simulink library "Library_Betriebsstrategie"  (R2018b)
settings: Solver=VariableStepAuto  StartTime=0.0  StopTime=10.0  RelTol=1e-3  EnableMultiTasking=on
undefined symbols (not defined in the file): akt_eUELG_HA, akt_eUELG_VA, akt_keinMVS_HA, akt_keinMVS_VA, akt_LSD_HA, akt_LSD_VA, akt_mUELG_HA, akt_mUELG_VA, akt_OD_HA, akt_OD_VA, DiscIntNeverNeededParam, magnitude, mu_road, mu_road_LF, mu_road_LR, mu_road_RF, mu_road_RR, par_MDT, par_VEH, stepsize
libraries: simulink x13
(part 1 of 6)
settings Model: Creator=ga76fur  LastModifiedBy=ga35gug
settings DataIOCC: LimitDataPoints=on
settings OptimizationCC: LifeSpan=inf
settings DebuggingCC: AllowSymbolicDim=off  SFUnexpectedBacktrackingDiag=warning  SFNoUnconditionalDefaultTransitionDiag=warning  SFExecutionAtInitializationDiag=none
settings ModelReferenceCC: PropagateSignalLabelsOutOfModel=off
settings SFSimCC: SimUseLocalCustomCode=off
settings RTWCC: RTWUseLocalCustomCode=off
settings CodeAppCC: StateflowObjectComments=on
settings GRTTargetCC: TargetLangStandard=C89/C90 (ANSI)
settings ConfigComp: CovMetricSettings=dw  CovHtmlReporting=on  CovSaveCumulativeToWorkspaceVar=on  CovSaveSingleToWorkspaceVar=on  CovExternalEMLEnable=off

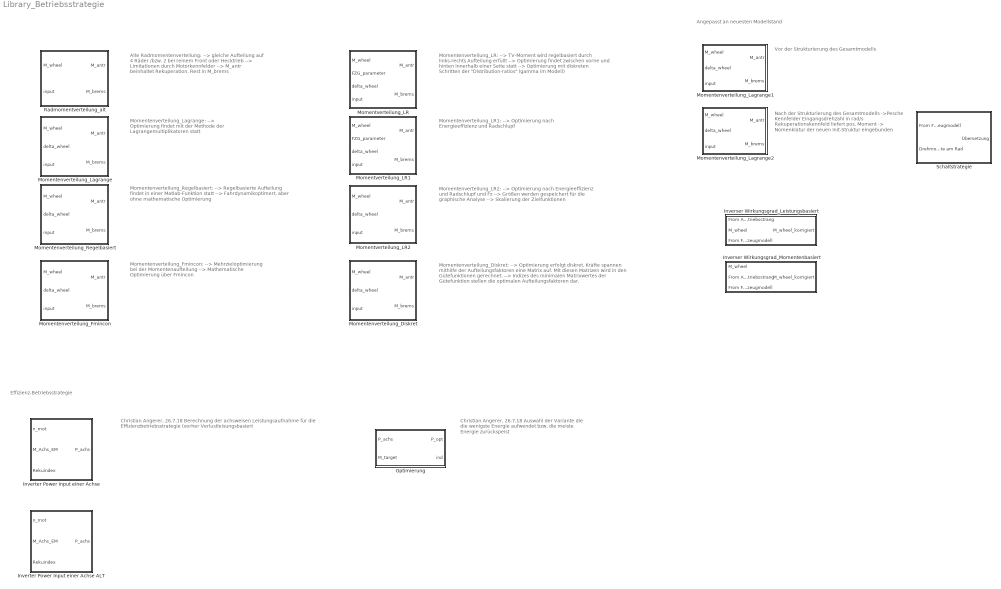
== system Library_Betriebsstrategie ==
  note: Effizienz-Betriebsstrategie
  note: Christian Angerer, 26.7.18
      | Berechnung der achsweisen Leistungsaufnahme für die Effizienzbetriebsstrategie
      | (vorher Verlustleisungsbasiert
  note: Nach der Strukturierung des Gesamtmodells
      | ->Pesche Kennfelder
      | 	Eingangsdrehzahl in rad/s
      | 	Rekuperationskennfeld liefert pos. Moment
      | -> Nomenklatur der neuen Init-Struktur eingebunden
  note: Vor der Strukturierung des Gesamtmodells
  note: Angepasst an neuesten Modellstand
  note: Momentenverteilung_Lagrange:
      | --> Optimierung findet mit der Methode der
      | 	Lagrangemultiplikatoren statt
  note: Momentenverteilung_LR1:
      | --> Optimierung nach Energieeffizienz und Radschlupf
  note: Momentenverteilung_Diskret:
      | --> Optimierung erfolgt diskret. Kräfte spannen mithilfe der
      | 	Aufteilungsfaktoren eine Matrix auf. Mit diesen Matrizen wird in den 		Gütefunktionen gerechnet.
      | --> Indizes des minimalen Matrixwertes der Gütefunktion stellen die 			optimalen Aufteilungsfaktoren dar.
  note: Momentenverteilung_Fmincon:
      | --> Mehrzieloptimierung bei der Momentenaufteilung
      | --> Mathematische Optimierung über Fmincon
  note: Momentenverteilung_Regelbasiert:
      | --> Regelbasierte Aufteilung findet in einer Matlab-Funktion statt
      | --> Fahrdynamikoptimert, aber ohne mathematische Optimierung
  note: Momentenverteilung_LR:
      | --> TV-Moment wird regelbasiert durch links-rechts Aufteilung erfüllt
      | --> Optimierung findet zwischen vorne und hinten
      | innerhalb einer Seite statt
      | --> Optimierung mit diskreten Schritten der "Distribution-ratios"
      | (gamma im Modell)
  note: Alte Radmomentenverteilung:
      | --> gleiche Aufteilung auf 4 Räder
      |     /bzw. 2 bei reinem Front oder Hecktrieb
      | --> Limitationen durch Motorkennfelder
      | --> M_antr beinhaltet Rekuperation, Rest in M_brems
  note: Momentenverteilung_LR2:
      | --> Optimierung nach Energieeffizienz und Radschlupf und Fz
      | --> Größen werden gespeichert für die graphische Analyse
      | --> Skalierung der Zielfunktionen
  note: Christian Angerer, 26.7.18
      | Auswahl der Variante die die wenigste Energie
      | aufwendet bzw. die meiste Energie zurückspeist
  Inverser Wirkungsgrad_Leistungsbasiert : Subsystem
  Inverser Wirkungsgrad_Momentenbasiert : Subsystem
  Inverter Power Input einer Achse : Subsystem  mask{U_RMS=par_MDT.VA.em.U_RMS, az=par_MDT.AUS.akt.az_VA, Powerfactor_map=par_MDT.VA.inv.Powerfactor_map, torque=par_MDT.VA.inv.torque, speed=par_MDT.VA.inv.speed, efficiency_map_LE=par_MDT.VA.inv.efficiency_map.efficiency_map_LE, current=par_MDT.VA.inv.current, voltage=par_MDT.VA.inv.voltage, powerfactor=par_MDT.VA.inv.powerfactor, MotorEffMap3D=par_MDT.VA.em.MotorEffMap3D, MotorEffMap3D_w=par_MDT.VA.em.MotorEffMap3D_w, MotorEffMap3D_M=par_MDT.VA.em.MotorEffMap3D_M, GeneratorEffMap3D=par_MDT.VA.em.GeneratorEffMap3D, GeneratorEffMap3D_w=par_MDT.VA.em.GeneratorEffMap3D_w, GeneratorEffMap3D_M=par_MDT.VA.em.GeneratorEffMap3D_M}
      mask prompts: U_RMS "RMS-Spannung"; az "Achszentrale Konfiguration"; Powerfactor_map "Map"; torque "torque-vector"; speed "speed-vector"; efficiency_map_LE "Map"; current "Stromvektor"; voltage "Spannungsvektor"; powerfactor "Powerfactor-Vektor"; MotorEffMap3D "Map"; MotorEffMap3D_w "Omega-Vektor"; MotorEffMap3D_M "Momenten-Vektor"; GeneratorEffMap3D "Map"; GeneratorEffMap3D_w "Omega-Vektor"; GeneratorEffMap3D_M "Momenten-Vektor"
      mask DialogControl Container3 Prompt: Einzelwerte
      mask DialogControl ParameterGroupVar Prompt: Powerfactor-Map
      mask DialogControl Container4 Prompt: LE-Efficiency Map
      mask DialogControl Container5 Prompt: Motor-Efficiency Maps
      mask DialogControl Container6 Prompt: Gen-Efficiency Maps
  Inverter Power Input einer Achse ALT : Subsystem  mask{U_RMS=par_MDT.VA.em.U_RMS, az=par_MDT.AUS.akt.az_VA, Powerfactor_map=par_MDT.VA.inv.Powerfactor_map, torque=par_MDT.VA.inv.torque, speed=par_MDT.VA.inv.speed, efficiency_map_LE=par_MDT.VA.inv.efficiency_map.efficiency_map_LE, current=par_MDT.VA.inv.current, voltage=par_MDT.VA.inv.voltage, powerfactor=par_MDT.VA.inv.powerfactor, MotorEffMap3D=par_MDT.VA.em.MotorEffMap3D, MotorEffMap3D_w=par_MDT.VA.em.MotorEffMap3D_w, MotorEffMap3D_M=par_MDT.VA.em.MotorEffMap3D_M, GeneratorEffMap3D=par_MDT.VA.em.GeneratorEffMap3D, GeneratorEffMap3D_w=par_MDT.VA.em.GeneratorEffMap3D_w, GeneratorEffMap3D_M=par_MDT.VA.em.GeneratorEffMap3D_M}
      mask prompts: U_RMS "RMS-Spannung"; az "Achszentrale Konfiguration"; Powerfactor_map "Map"; torque "torque-vector"; speed "speed-vector"; efficiency_map_LE "Map"; current "Stromvektor"; voltage "Spannungsvektor"; powerfactor "Powerfactor-Vektor"; MotorEffMap3D "Map"; MotorEffMap3D_w "Omega-Vektor"; MotorEffMap3D_M "Momenten-Vektor"; GeneratorEffMap3D "Map"; GeneratorEffMap3D_w "Omega-Vektor"; GeneratorEffMap3D_M "Momenten-Vektor"
      mask DialogControl Container3 Prompt: Einzelwerte
      mask DialogControl ParameterGroupVar Prompt: Powerfactor-Map
      mask DialogControl Container4 Prompt: LE-Efficiency Map
      mask DialogControl Container5 Prompt: Motor-Efficiency Maps
      mask DialogControl Container6 Prompt: Gen-Efficiency Maps
  Momentenverteilung_Diskret : Subsystem
  Momentenverteilung_Fmincon : Subsystem
  Momentenverteilung_Lagrange : Subsystem
  Momentenverteilung_Lagrange1 : Subsystem
  Momentenverteilung_Lagrange2 : Subsystem
  Momentenverteilung_Regelbasiert : Subsystem
  Momentverteilung_LR : Subsystem
  Momentverteilung_LR1 : Subsystem
  Momentverteilung_LR2 : Subsystem
  Optimierung : MATLAB Function  TreatAsAtomicUnit=on
  Radmomentverteilung_alt : Subsystem
  Schaltstrategie : Subsystem

== system Library_Betriebsstrategie/Inverser Wirkungsgrad_Leistungsbasiert ==
  note: Das Modell berücksichtigt nun einen verlustbehafteten Antriebsstrang vor dem Fahrzeugmodell.
      | --> Der Inverse Gesamtwirkungsgrad des vorherigen Zeitschrittes wird auf das Gesamtwunschmoment aufmultipliziert.
      | eta=P_ab/(P_ab+P_v)
  From Antriebsstrang : Inport
  M_wheel : Inport  Port=2
  From Fahrzeugmodell : Inport  Port=3
  1 : Constant
  Abs : Abs
  Abs1 : Abs
  Add : Sum
  Divide : Product  Inputs=/*
  Divide1 : Product  Inputs=/*
  Eins : Constant
  Memory : Memory
  Memory1 : Memory
  Product : Product
  Scope : Scope  NumInputPorts=2
  Scope1 : Scope  NumInputPorts=2
  Switch : Switch  Criteria=u2 > Threshold  Threshold=0.1
  M_wheel_korrigiert : Outport
  wires:
  Product/1 -> Scope1/1, M_wheel_korrigiert/1
  Eins/1 -> Divide/2
  Add/1 -> Switch/2, Divide1/1
  From Antriebsstrang/1 -> Scope/1, Memory/1
  Divide1/1 -> Divide/1
  Memory/1 -> Abs/1
  Memory1/1 -> Abs1/1
  Divide/1 -> Switch/1
  M_wheel/1 -> Scope1/2, Product/2
  Switch/1 -> Product/1
  1/1 -> Switch/3
  Abs/1 -> Add/1
  Abs1/1 -> Add/2, Divide1/2
  From Fahrzeugmodell/1 -> ?
  ? -> Scope/2, Memory1/1

== system Library_Betriebsstrategie/Inverser Wirkungsgrad_Momentenbasiert ==
  M_wheel : Inport
  From Antriebsstrang : Inport  Port=2
  From Fahrzeugmodell : Inport  Port=3
  1 : Constant
  Abs : Abs
  Abs1 : Abs
  Add1 : Sum  Inputs=++++
  Divide : Product  Inputs=/*
  Memory : Memory
  Memory1 : Memory
  Product : Product
  Scope : Scope  NumInputPorts=2
  Scope1 : Scope  NumInputPorts=2
  Switch : Switch  Criteria=u2 > Threshold
  M_wheel_korrigiert : Outport
  wires:
  Product/1 -> Scope/1, M_wheel_korrigiert/1
  M_wheel/1 -> Scope1/1, Memory1/1, Scope/2, Product/2
  Add1/1 -> Scope1/2, Memory/1
  Memory/1 -> Abs/1
  Memory1/1 -> Abs1/1
  Switch/1 -> Product/1
  1/1 -> Switch/3
  Abs1/1 -> Divide/2
  From Antriebsstrang/1 -> ?
  ? -> Add1/1
  ? -> Add1/2
  ? -> Add1/3
  ? -> Add1/4
  Abs/1 -> Switch/2, Divide/1
  Divide/1 -> Switch/1

== system Library_Betriebsstrategie/Inverter Power Input einer Achse ==
  note: Luca Mantovani, 05.9.18
      | Power estimation for electronics and motor is calculated with the same logic as found in Antriebsstrang una Radmomentverteilung. The electric power entering the motor is evaluated first and with the result the power at battery level is found.
  n_mot : Inport
  M_Achs_EM : Inport  Port=2
  Rekuindex : Inport  Port=3
  Abs{1..2,4..6} (5 alike) : Abs
  Constant1 : Constant  Value=U_RMS
  "Falls radnahe Maschine " : Subsystem
  Falls radnahe Maschine 1 : Subsystem
  Gain : Gain  Gain=-1
  Gain2 : Gain  Gain=-1
  Math Function : Math  Operator=pow  SaturateOnIntegerOverflow=on
  Math Function1 : Math  Operator=pow  SaturateOnIntegerOverflow=on
  Powerfactorberechnung : Subsystem
  Product1 : Product  Inputs=**
  Product3 : Product  Inputs=**
  Product5 : Product  Inputs=**
  Sign : Signum
  Stromberechnung : Subsystem
  W-->kW : Gain  Gain=0.001
  Wirkungsgradberechnung : Subsystem
  Wirkungsgradberechnung1 : Subsystem
  P_achs : Outport
  wires:
  Product1/1 -> Product3/1
  Abs6/1 -> Falls radnahe Maschine 1/1(M_achs_EM)
  W-->kW/1 -> P_achs/1
  Math Function/1 -> Product3/2
  Product5/1 -> Abs6/1  "P_inverter"
  M_Achs_EM/1 -> "Falls radnahe Maschine "/1(M_achs_EM)
  Product3/1 -> Abs2/1, Sign/1, Product5/2  "P_EM"
  Gain/1 -> Math Function/2
  Wirkungsgradberechnung/1(Wirkungsgrad EM) -> Math Function/1
  Rekuindex/1 -> Gain/1
  "Falls radnahe Maschine "/1(M_mot) -> Product1/2, Abs4/1, Wirkungsgradberechnung/2(M_mot)
  Abs2/1 -> Stromberechnung/1(Leistung)
  Wirkungsgradberechnung1/1(Wirkungsgrad_LE) -> Math Function1/1
  Abs5/1 -> Powerfactorberechnung/2(Drehzahl)
  Abs4/1 -> Powerfactorberechnung/1(Drehmoment)
  Powerfactorberechnung/1(Powerfactor) -> Stromberechnung/3(Powerfactor), Wirkungsgradberechnung1/3(Powerfactor)
  n_mot/1 -> Product1/1, Abs1/1, Abs5/1
  Sign/1 -> Gain2/1
  Gain2/1 -> Math Function1/2
  Constant1/1 -> Stromberechnung/2(Spannung), Wirkungsgradberechnung1/2(Spannung)
  Stromberechnung/1(Strom) -> Wirkungsgradberechnung1/1(Strom)
  Math Function1/1 -> Product5/1
  Abs1/1 -> Wirkungsgradberechnung/1(n_mot)
  Falls radnahe Maschine 1/1(M_mot) -> W-->kW/1

== system Library_Betriebsstrategie/Inverter Power Input einer Achse ALT ==
  n_mot : Inport
  M_Achs_EM : Inport  Port=2
  Rekuindex : Inport  Port=3
  Abs : Abs
  Abs6 : Abs
  Add1 : Sum
  Constant2 : Constant  Value=U_RMS
  "Falls radnahe Maschine " : Subsystem
  Leistungselektronik : Subsystem
  Product1 : Product  Inputs=**
  Product3 : Product  Inputs=**
  Product5 : Product  Inputs=**
  W-->kW : Gain  Gain=0.001
  Wirkungsgradberechnung : Subsystem
  P_achs : Outport
  wires:
  Product1/1 -> Product3/1, Product5/2
  Abs/1 -> Add1/2
  Abs6/1 -> Add1/1
  Add1/1 -> W-->kW/1
  W-->kW/1 -> P_achs/1
  Constant2/1 -> Leistungselektronik/1(RMS Spannung)
  "Falls radnahe Maschine "/1(M_mot) -> Leistungselektronik/2(Drehmoment_1EM), Wirkungsgradberechnung/2(M_mot)
  Wirkungsgradberechnung/1(Wirkungsgrad EM) -> Product3/2
  Leistungselektronik/1(Verlustgrad LE) -> Product5/1
  Rekuindex/1 -> Wirkungsgradberechnung/3(Rekuindex)
  Product5/1 -> Abs6/1  "P_loss_inverter"
  Product3/1 -> Abs/1  "P_EM"
  M_Achs_EM/1 -> "Falls radnahe Maschine "/1(M_achs_EM), Product1/2
  n_mot/1 -> Product1/1, Wirkungsgradberechnung/1(n_mot), Leistungselektronik/3("Drehzahl ")

== system Library_Betriebsstrategie/Momentenverteilung_Diskret ==
  M_wheel : Inport
  delta_wheel : Inport  Port=2
  input : Inport  Port=3
  Bus Selector3 : BusSelector  OutputSignals=x.vx
  Constant1 : Constant  Value=par_VEH.bkv
  Feedback Controller : Subsystem
  Gierrate Referenz Berechnung : Subsystem
  Memory : Memory
  Momente für die Reibbremse : Subsystem
  Radmomentenaufteilung : Subsystem
  Scope : Scope  NumInputPorts=2
  M_antr : Outport
  M_brems : Outport  Port=2
  wires:
  delta_wheel/1 -> Gierrate Referenz Berechnung/2(delta_wheel)
  input/1 -> Memory/1
  Feedback Controller/1(M_z_desired) -> Radmomentenaufteilung/2(M_z_desired), Scope/1  "M_z_desired"
  Gierrate Referenz Berechnung/1(Gierrate ref) -> Feedback Controller/2(Gierrate ref)  "psip_ref"
  Radmomentenaufteilung/1(M_antr) -> M_antr/1, Momente für die Reibbremse/1(M_antr)
  Momente für die Reibbremse/1(M_brems) -> M_brems/1
  M_wheel/1 -> Momente für die Reibbremse/2(M_wheel), Radmomentenaufteilung/3(M_wheel), Scope/2
  Bus Selector3/1 -> Momente für die Reibbremse/3(v_x)  "<vx>"
  Memory/1 -> Gierrate Referenz Berechnung/1(input), Feedback Controller/1(Input), Radmomentenaufteilung/1(Input), Bus Selector3/1
  Constant1/1 -> Momente für die Reibbremse/4(bkv)

== system Library_Betriebsstrategie/Momentenverteilung_Fmincon ==
  M_wheel : Inport
  delta_wheel : Inport  Port=2
  input : Inport  Port=3
  Bus Selector3 : BusSelector  OutputSignals=x.vx
  Constant1 : Constant  Value=par_VEH.bkv
  Feedback Controller : Subsystem
  Gierrate Referenz Berechnung : Subsystem
  Limitierungen gesamt : Subsystem
  Memory : Memory
  Momente für die Reibbremse : Subsystem
  Motor Limits : Subsystem
  Radmomentenaufteilung : Subsystem
  Reifen Limits : Subsystem
  M_antr : Outport
  M_brems : Outport  Port=2
  wires:
  delta_wheel/1 -> Gierrate Referenz Berechnung/2(delta_wheel)
  input/1 -> Memory/1
  Feedback Controller/1(M_z_desired) -> Radmomentenaufteilung/3(M_z_desired)  "M_z_desired"
  Gierrate Referenz Berechnung/1(Gierrate ref) -> Feedback Controller/2(Gierrate ref)  "psip_ref"
  Radmomentenaufteilung/1(M_antr) -> M_antr/1, Momente für die Reibbremse/1(M_antr)
  Momente für die Reibbremse/1(M_brems) -> M_brems/1
  M_wheel/1 -> Momente für die Reibbremse/2(M_wheel), Radmomentenaufteilung/4(M_wheel)
  Bus Selector3/1 -> Momente für die Reibbremse/3(v_x)  "<vx>"
  Reifen Limits/1(Fx_limit) -> Limitierungen gesamt/1(Fx_limit)
  Motor Limits/1(M_limit) -> Limitierungen gesamt/2(M_limit)
  Memory/1 -> Reifen Limits/1(Input), Motor Limits/1(Input), Feedback Controller/1(Input), Bus Selector3/1, Radmomentenaufteilung/2(Input), Gierrate Referenz Berechnung/1(input)
  Limitierungen gesamt/1(Fx_limits) -> Radmomentenaufteilung/1(Fx_limits)
  Constant1/1 -> Momente für die Reibbremse/4(bkv)

== system Library_Betriebsstrategie/Momentenverteilung_Lagrange ==
  M_wheel : Inport
  delta_wheel : Inport  Port=2
  input : Inport  Port=3
  Bus Selector3 : BusSelector  OutputSignals=x.vx
  Feedback Controller : Subsystem
  Gierrate Referenz Berechnung : Subsystem
  Memory : Memory
  Momente für die Reibbremse : Subsystem
  Radmomentenaufteilung : Subsystem
  M_antr : Outport
  M_brems : Outport  Port=2
  wires:
  delta_wheel/1 -> Gierrate Referenz Berechnung/2(delta_wheel), Radmomentenaufteilung/4(Delta_wheel)
  input/1 -> Memory/1
  Feedback Controller/1(M_z_desired) -> Radmomentenaufteilung/2(M_z_desired)  "M_z_desired"
  Gierrate Referenz Berechnung/1(Gierrate ref) -> Feedback Controller/2(Gierrate ref)  "psip_ref"
  Radmomentenaufteilung/1(M_antr) -> M_antr/1, Momente für die Reibbremse/1(M_antr)
  Momente für die Reibbremse/1(M_brems) -> M_brems/1
  M_wheel/1 -> Momente für die Reibbremse/2(M_wheel), Radmomentenaufteilung/3(M_wheel)
  Bus Selector3/1 -> Momente für die Reibbremse/3(v_x)  "<vx>"
  Memory/1 -> Feedback Controller/1(Input), Bus Selector3/1, Radmomentenaufteilung/1(Input), Gierrate Referenz Berechnung/1(input)

== system Library_Betriebsstrategie/Momentenverteilung_Lagrange1 ==
  M_wheel : Inport
  delta_wheel : Inport  Port=2
  input : Inport  Port=3
  Bus Selector3 : BusSelector  OutputSignals=x.vx
  Feedback Controller : Subsystem
  Gierrate Referenz Berechnung : Subsystem
  Limitierungen gesamt (mit MVS Limits) : Subsystem
  Memory : Memory
  Momente für die Reibbremse : Subsystem
  Motor Limits : Subsystem
  Radmomentenaufteilung : Subsystem
  Reifen Limits : Subsystem
  Scope : Scope  NumInputPorts=2
  M_antr : Outport
  M_brems : Outport  Port=2
  wires:
  Bus Selector3/1 -> Momente für die Reibbremse/3(v_x)  "<vx>"
  M_wheel/1 -> Radmomentenaufteilung/4(M_wheel), Momente für die Reibbremse/2(M_wheel), Scope/2
  Momente für die Reibbremse/1(M_brems) -> M_brems/1
  Radmomentenaufteilung/1(M_antr) -> M_antr/1, Momente für die Reibbremse/1(M_antr)
  Gierrate Referenz Berechnung/1(Gierrate ref) -> Feedback Controller/2(Gierrate ref)  "psip_ref"
  Feedback Controller/1(M_z_desired) -> Radmomentenaufteilung/3(M_z_desired), Scope/1  "M_z_desired"
  input/1 -> Memory/1
  delta_wheel/1 -> Radmomentenaufteilung/5(Delta_wheel), Gierrate Referenz Berechnung/2(delta_wheel)
  Motor Limits/2(M_limit_zentral) -> Limitierungen gesamt (mit MVS Limits)/3(M_limit_zentral)
  Memory/1 -> Gierrate Referenz Berechnung/1(input), Bus Selector3/1, Radmomentenaufteilung/2(Input), Feedback Controller/1(Input), Motor Limits/1(Input), Reifen Limits/1(Input)
  Motor Limits/1(M_limit) -> Limitierungen gesamt (mit MVS Limits)/2(M_limit)
  Reifen Limits/1(Fx_limit) -> Limitierungen gesamt (mit MVS Limits)/1(Fx_limit)
  Limitierungen gesamt (mit MVS Limits)/1(Fx_limits) -> Radmomentenaufteilung/1(Fx_limits)

== system Library_Betriebsstrategie/Momentenverteilung_Lagrange2 ==
  M_wheel : Inport
  delta_wheel : Inport  Port=2
  input : Inport  Port=3
  Bus Selector3 : BusSelector  OutputSignals=x.vx
  Feedback Controller : Subsystem
  Gierrate Referenz Berechnung : Subsystem
  Limitierungen gesamt (mit MVS Limits) : Subsystem
  Memory : Memory
  Momente für die Reibbremse : Subsystem
  Motor Limits : Subsystem
  Radmomentenaufteilung1 : Subsystem
  Reifen Limits : Subsystem
  Scope : Scope  NumInputPorts=2
  M_antr : Outport
  M_brems : Outport  Port=2
  wires:
  Limitierungen gesamt (mit MVS Limits)/1(Fx_limits) -> Radmomentenaufteilung1/1(Fx_limits)
  Reifen Limits/1(Fx_limit) -> Limitierungen gesamt (mit MVS Limits)/1(Fx_limit)
  Motor Limits/1(M_limit) -> Limitierungen gesamt (mit MVS Limits)/2(M_limit)
  Memory/1 -> Motor Limits/1(Input), Reifen Limits/1(Input), Feedback Controller/1(Input), Bus Selector3/1, Radmomentenaufteilung1/2(Input), Gierrate Referenz Berechnung/1(input)
  Motor Limits/2(M_limit_zentral) -> Limitierungen gesamt (mit MVS Limits)/3(M_limit_zentral)
  delta_wheel/1 -> Radmomentenaufteilung1/5(Delta_wheel), Gierrate Referenz Berechnung/2(delta_wheel)
  input/1 -> Memory/1
  Feedback Controller/1(M_z_desired) -> Radmomentenaufteilung1/3(M_z_desired), Scope/1  "M_z_desired"
  Gierrate Referenz Berechnung/1(Gierrate ref) -> Feedback Controller/2(Gierrate ref)  "psip_ref"
  Radmomentenaufteilung1/1(M_antr) -> M_antr/1, Momente für die Reibbremse/1(M_antr)
  Momente für die Reibbremse/1(M_brems) -> M_brems/1
  M_wheel/1 -> Scope/2, Radmomentenaufteilung1/4(M_wheel), Momente für die Reibbremse/2(M_wheel)
  Bus Selector3/1 -> Momente für die Reibbremse/3(v_x)  "<vx>"

== system Library_Betriebsstrategie/Momentenverteilung_Regelbasiert ==
  M_wheel : Inport
  delta_wheel : Inport  Port=2
  input : Inport  Port=3
  Bus Selector3 : BusSelector  OutputSignals=x.vx
  Constant10 : Constant  Value=par_VEH.bkv
  Feedback Controller : Subsystem
  Gierrate Referenz Berechnung : Subsystem
  Limitierungen gesamt : Subsystem
  Memory : Memory
  Momente für die Reibbremse : Subsystem
  Motor Limits : Subsystem
  Radmomentenaufteilung : Subsystem
  Reifen Limits : Subsystem
  M_antr : Outport
  M_brems : Outport  Port=2
  wires:
  delta_wheel/1 -> Gierrate Referenz Berechnung/2(delta_wheel)
  input/1 -> Memory/1
  Feedback Controller/1(M_z_desired) -> Radmomentenaufteilung/4(M_z_desired)  "M_z_desired"
  Gierrate Referenz Berechnung/1(Gierrate ref) -> Feedback Controller/2(Gierrate ref)  "psip_ref"
  Radmomentenaufteilung/1(M_antr) -> Momente für die Reibbremse/1(M_antr), M_antr/1
  Momente für die Reibbremse/1(M_brems) -> M_brems/1
  M_wheel/1 -> Momente für die Reibbremse/2(M_wheel), Radmomentenaufteilung/3(M_wheel)
  Bus Selector3/1 -> Momente für die Reibbremse/3(v_x)  "<vx>"
  Memory/1 -> Gierrate Referenz Berechnung/1(input), Reifen Limits/1(Input), Motor Limits/1(Input), Feedback Controller/1(Input), Bus Selector3/1, Radmomentenaufteilung/2(Input)
  Motor Limits/1(M_limit) -> Limitierungen gesamt/2(M_limit)
  Limitierungen gesamt/1(Fx_limits) -> Radmomentenaufteilung/1(Fx_limits)
  Constant10/1 -> Momente für die Reibbremse/4(bkv)
  Reifen Limits/1(Fx_limit) -> Limitierungen gesamt/1(Fx_limit)

== system Library_Betriebsstrategie/Momentverteilung_LR ==
  M_wheel : Inport
  FZG_parameter : Inport  Port=2
  delta_wheel : Inport  Port=3
  input : Inport  Port=4
  Bus Creator : BusCreator  Inputs=4
  Bus Creator1 : BusCreator  Inputs=4
  Bus Selector1 : BusSelector  OutputSignals=Iz
  Bus Selector2 : BusSelector  OutputSignals=psi.psip
  Bus Selector3 : BusSelector  OutputSignals=x.vx
  Bus Selector4 : BusSelector  OutputSignals=bkv
  Feedback Controller : Subsystem
  Gierrate Referenz Berechnung : Subsystem
  Memory : Memory
  Momente für die Reibbremse : Subsystem
  Motor Limits : Subsystem
  Radmomentenaufteilung : Subsystem
  Reifen Limits : Subsystem
  M_antr : Outport
  M_brems : Outport  Port=2
  wires:
  FZG_parameter/1 -> Bus Selector1/1, Radmomentenaufteilung/4(FZG parameter), Bus Selector4/1, Gierrate Referenz Berechnung/3(FZG parameter)
  delta_wheel/1 -> Gierrate Referenz Berechnung/2(delta_wheel)
  input/1 -> Memory/1
  Feedback Controller/1(M_z_desired) -> Radmomentenaufteilung/3(M_z_desired)  "M_z_desired"
  Gierrate Referenz Berechnung/1(Gierrate ref) -> Feedback Controller/2(Gierrate ref)  "psip_ref"
  Bus Selector2/1 -> Feedback Controller/1(Gierrate)  "<psip>"
  Radmomentenaufteilung/1(M_antr_LF) -> Bus Creator/1  "M_antr_LF"
  Radmomentenaufteilung/4(M_antr_RR) -> Bus Creator/4  "M_antr_RR"
  Radmomentenaufteilung/3(M_antr_RF) -> Bus Creator/3  "M_antr_RF"
  Radmomentenaufteilung/2(M_antr_LR) -> Bus Creator/2  "M_antr_LR"
  Bus Selector1/1 -> Feedback Controller/3(Iz)  "<Iz>"
  Bus Creator/1 -> Momente für die Reibbremse/1(M_antr), M_antr/1
  Bus Creator1/1 -> M_brems/1
  M_wheel/1 -> Momente für die Reibbremse/2(M_wheel), Radmomentenaufteilung/2(M_wheel)
  Momente für die Reibbremse/1(LF) -> Bus Creator1/1  "M_brems_LF"
  Momente für die Reibbremse/2(LR) -> Bus Creator1/2  "M_brems_LR"
  Momente für die Reibbremse/3(RF) -> Bus Creator1/3  "M_brems_RF"
  Momente für die Reibbremse/4(RR) -> Bus Creator1/4  "M_brems_RR"
  Bus Selector4/1 -> Momente für die Reibbremse/4(bkv)  "<bkv>"
  Bus Selector3/1 -> Momente für die Reibbremse/3(v_x)  "<vx>"
  Memory/1 -> Bus Selector2/1, Bus Selector3/1, Radmomentenaufteilung/1(Input), Motor Limits/1(Input), Gierrate Referenz Berechnung/1(input)

== system Library_Betriebsstrategie/Momentverteilung_LR1 ==
  M_wheel : Inport
  FZG_parameter : Inport  Port=2
  delta_wheel : Inport  Port=3
  input : Inport  Port=4
  Bus Creator : BusCreator  Inputs=4
  Bus Creator1 : BusCreator  Inputs=4
  Bus Selector1 : BusSelector  OutputSignals=Iz
  Bus Selector2 : BusSelector  OutputSignals=psi.psip
  Bus Selector3 : BusSelector  OutputSignals=x.vx
  Bus Selector4 : BusSelector  OutputSignals=bkv
  Feedback Controller : Subsystem
  Gierrate Referenz Berechnung : Subsystem
  Limitierungen gesamt : Subsystem
  Memory : Memory
  Momente für die Reibbremse : Subsystem
  Momentenverteilende Systeme Limits : Subsystem
  Motor Limits : Subsystem
  Radmomentenaufteilung : Subsystem
  Reifen Limits : Subsystem
  M_antr : Outport
  M_brems : Outport  Port=2
  wires:
  Bus Selector3/1 -> Momente für die Reibbremse/3(v_x)  "<vx>"
  Bus Selector4/1 -> Momente für die Reibbremse/4(bkv)  "<bkv>"
  Momente für die Reibbremse/4(RR) -> Bus Creator1/4  "M_brems_RR"
  Momente für die Reibbremse/3(RF) -> Bus Creator1/3  "M_brems_RF"
  Momente für die Reibbremse/2(LR) -> Bus Creator1/2  "M_brems_LR"
  Momente für die Reibbremse/1(LF) -> Bus Creator1/1  "M_brems_LF"
  M_wheel/1 -> Radmomentenaufteilung/2(M_wheel), Momente für die Reibbremse/2(M_wheel)
  Bus Creator1/1 -> M_brems/1
  Bus Creator/1 -> M_antr/1, Momente für die Reibbremse/1(M_antr)
  Bus Selector1/1 -> Feedback Controller/3(Iz)  "<Iz>"
  Radmomentenaufteilung/2(M_antr_LR) -> Bus Creator/2  "M_antr_LR"
  Radmomentenaufteilung/3(M_antr_RF) -> Bus Creator/3  "M_antr_RF"
  Radmomentenaufteilung/4(M_antr_RR) -> Bus Creator/4  "M_antr_RR"
  Radmomentenaufteilung/1(M_antr_LF) -> Bus Creator/1  "M_antr_LF"
  Bus Selector2/1 -> Feedback Controller/1(Gierrate)  "<psip>"
  Gierrate Referenz Berechnung/1(Gierrate ref) -> Feedback Controller/2(Gierrate ref)  "psip_ref"
  Feedback Controller/1(M_z_desired) -> Radmomentenaufteilung/3(M_z_desired)  "M_z_desired"
  input/1 -> Memory/1
  delta_wheel/1 -> Gierrate Referenz Berechnung/2(delta_wheel)
  FZG_parameter/1 -> Gierrate Referenz Berechnung/3(FZG parameter), Bus Selector4/1, Radmomentenaufteilung/4(FZG parameter), Bus Selector1/1
  Momentenverteilende Systeme Limits/1(MVS_limit) -> Limitierungen gesamt/3(MVS_limit)
  Reifen Limits/1(Fx_limit) -> Limitierungen gesamt/1(Fx_limit)
  Motor Limits/1(M_limit) -> Limitierungen gesamt/2(M_limit)
  Memory/1 -> Gierrate Referenz Berechnung/1(input), Momentenverteilende Systeme Limits/1(Input), Motor Limits/1(Input), Reifen Limits/1(Input), Radmomentenaufteilung/1(Input), Bus Selector3/1, Bus Selector2/1

== system Library_Betriebsstrategie/Momentverteilung_LR2 ==
  M_wheel : Inport
  delta_wheel : Inport  Port=2
  input : Inport  Port=3
  Bus Creator : BusCreator  Inputs=4
  Bus Creator1 : BusCreator  Inputs=4
  Bus Selector2 : BusSelector  OutputSignals=psi.psip
  Bus Selector3 : BusSelector  OutputSignals=x.vx
  Constant10 : Constant  Value=par_VEH.bkv
  Feedback Controller : Subsystem
  Gierrate Referenz Berechnung : Subsystem
  Limitierungen gesamt (mit MVS Limits) : Subsystem
  Memory : Memory
  Momente für die Reibbremse : Subsystem
  Motor Limits : Subsystem
  Radmomentenaufteilung : Subsystem
  Reifen Limits : Subsystem
  M_antr : Outport
  M_brems : Outport  Port=2
  wires:
  Motor Limits/2(M_limit_zentral) -> Limitierungen gesamt (mit MVS Limits)/3(M_limit_zentral)
  Memory/1 -> Gierrate Referenz Berechnung/1(input), Bus Selector2/1, Bus Selector3/1, Radmomentenaufteilung/1(Input), Motor Limits/1(Input), Reifen Limits/1(Input)
  Motor Limits/1(M_limit) -> Limitierungen gesamt (mit MVS Limits)/2(M_limit)
  Reifen Limits/1(Fx_limit) -> Limitierungen gesamt (mit MVS Limits)/1(Fx_limit)
  delta_wheel/1 -> Gierrate Referenz Berechnung/2(delta_wheel)
  input/1 -> Memory/1
  Feedback Controller/1(M_z_desired) -> Radmomentenaufteilung/3(M_z_desired)  "M_z_desired"
  Gierrate Referenz Berechnung/1(Gierrate ref) -> Feedback Controller/2(Gierrate ref)  "psip_ref"
  Bus Selector2/1 -> Feedback Controller/1(Gierrate)  "<psip>"
  Radmomentenaufteilung/1(M_antr_LF) -> Bus Creator/1  "M_antr_LF"
  Radmomentenaufteilung/4(M_antr_RR) -> Bus Creator/4  "M_antr_RR"
  Radmomentenaufteilung/3(M_antr_RF) -> Bus Creator/3  "M_antr_RF"
  Radmomentenaufteilung/2(M_antr_LR) -> Bus Creator/2  "M_antr_LR"
  Bus Creator/1 -> Momente für die Reibbremse/1(M_antr), M_antr/1
  Bus Creator1/1 -> M_brems/1
  M_wheel/1 -> Momente für die Reibbremse/2(M_wheel), Radmomentenaufteilung/2(M_wheel)
  Momente für die Reibbremse/1(LF) -> Bus Creator1/1  "M_brems_LF"
  Momente für die Reibbremse/2(LR) -> Bus Creator1/2  "M_brems_LR"
  Momente für die Reibbremse/3(RF) -> Bus Creator1/3  "M_brems_RF"
  Momente für die Reibbremse/4(RR) -> Bus Creator1/4  "M_brems_RR"
  Bus Selector3/1 -> Momente für die Reibbremse/3(v_x)  "<vx>"
  Constant10/1 -> Momente für die Reibbremse/4(bkv)

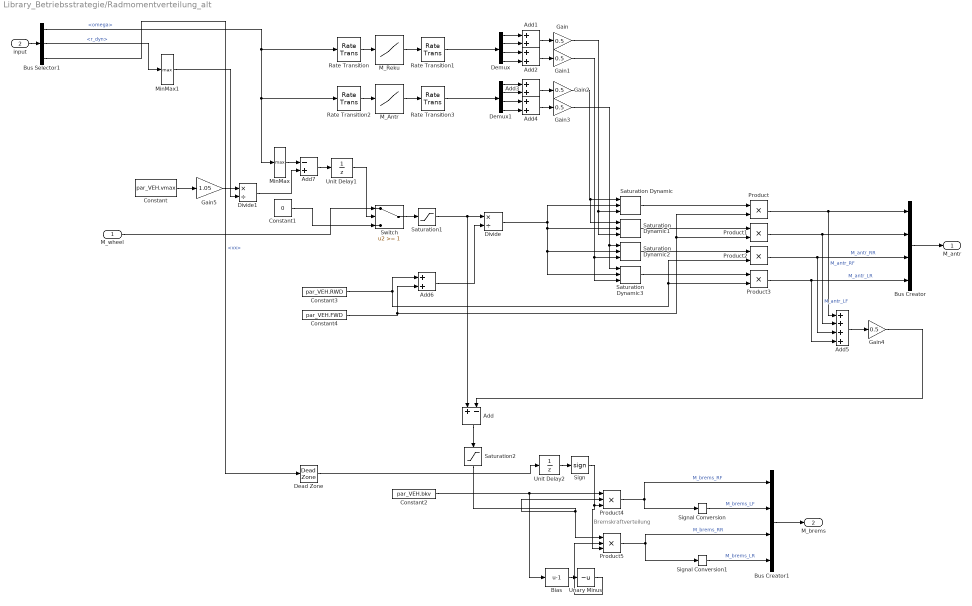
== system Library_Betriebsstrategie/Radmomentverteilung_alt ==
  note: Bremskraftverteilung
  M_wheel : Inport
  input : Inport  Port=2
  Add : Sum  Inputs=+-
  Add{1..4,6} (5 alike) : Sum
  Add5 : Sum  Inputs=++++
  Add7 : Sum  Inputs=-+
  Bias : Bias  Bias=-1
  Bus Creator : BusCreator  Inputs=4
  Bus Creator1 : BusCreator  Inputs=4
  Bus Selector1 : BusSelector  OutputSignals=omega,r_dyn,x.vx
  Constant : Constant  Value=par_VEH.vmax
  Constant1 : Constant  Value=0
  Constant2 : Constant  Value=par_VEH.bkv
  Constant3 : Constant  Value=par_VEH.RWD
  Constant4 : Constant  Value=par_VEH.FWD
  Dead Zone : DeadZone  LowerValue=-0.02  UpperValue=0.02  SaturateOnIntegerOverflow=on
  Demux : Demux
  Demux1 : Demux
  Divide : Product  Inputs=*/
  Divide1 : Product  Inputs=*/
  Gain{,1..4} (5 alike) : Gain  Gain=0.5
  Gain5 : Gain  Gain=1.05
  M_Antr : Lookup_n-D  NumberOfTableDimensions=1  BreakpointsForDimension1=par_VEH.dt_nmax/par_VEH.dt_i/60*2*pi  Table=par_VEH.dt_Mmax*par_VEH.dt_i/2  InternalRulePriority=Speed  RndMeth=Simplest  InputSameDT=on
  M_Reku : Lookup_n-D  NumberOfTableDimensions=1  BreakpointsForDimension1=par_VEH.dt_nmin/par_VEH.dt_i/60*2*pi  Table=par_VEH.dt_Mmin*par_VEH.dt_i/2  InternalRulePriority=Speed  RndMeth=Simplest  InputSameDT=on
  MinMax : MinMax  Function=max
  MinMax1 : MinMax  Function=max
  Product{,1..3} (4 alike) : Product
  Product4 : Product  Inputs=3
  Product5 : Product  Inputs=3
  Rate Transition : RateTransition  OutPortSampleTime=stepsize*10
  Rate Transition1 : RateTransition  OutPortSampleTimeOpt=Inherit  OutPortSampleTime=0.001
  Rate Transition2 : RateTransition  OutPortSampleTime=stepsize*10
  Rate Transition3 : RateTransition  OutPortSampleTimeOpt=Inherit  OutPortSampleTime=0.001
  Saturation Dynamic{,1..3} (4 alike) : simulink/Discontinuities/Saturation Dynamic  OutMin=[]  OutMax=[]  OutDataTypeStr=Inherit: Same as second input  OutDataType=fixdt(1, 16)  OutScaling=2^-10  DoSatur=off
  Saturation1 : Saturate  UpperLimit=1500  LowerLimit=-5000
  Saturation2 : Saturate  UpperLimit=0  LowerLimit=-5000
  Sign : Signum
  Signal Conversion : SignalConversion  OverrideOpt=off
  Signal Conversion1 : SignalConversion  OverrideOpt=off
  Switch : Switch  Threshold=1
  Unary Minus : UnaryMinus
  Unit Delay1 : UnitDelay  InitialCondition=2  SampleTime=-1
  Unit Delay2 : UnitDelay  InitialCondition=2  SampleTime=-1
  M_antr : Outport
  M_brems : Outport  Port=2
  wires:
  Product/1 -> Add5/1, Bus Creator/1  "M_antr_RF"
  Product1/1 -> Add5/2, Bus Creator/2  "M_antr_LF"
  Product2/1 -> Add5/3, Bus Creator/3  "M_antr_RR"
  Product3/1 -> Add5/4, Bus Creator/4  "M_antr_LR"
  M_Reku/1 -> Rate Transition1/1
  Rate Transition/1 -> M_Reku/1
  Add/1 -> Saturation2/1
  Saturation2/1 -> Product5/1, Product4/2
  Bus Creator/1 -> M_antr/1
  Bus Creator1/1 -> M_brems/1
  Constant2/1 -> Bias/1, Product4/1
  Bias/1 -> Unary Minus/1
  Unary Minus/1 -> Product5/2
  Signal Conversion/1 -> Bus Creator1/2  "M_brems_LF"
  Signal Conversion1/1 -> Bus Creator1/4  "M_brems_LR"
  M_Antr/1 -> Rate Transition3/1
  Rate Transition2/1 -> M_Antr/1
  Rate Transition1/1 -> Demux/1
  Demux/1 -> Add1/1
  Demux/2 -> Add1/2
  Add1/1 -> Gain/1
  Demux/3 -> Add2/1
  Demux/4 -> Add2/2
  Add2/1 -> Gain1/1
  Constant4/1 -> Product/2, Product1/2, Add6/2
  Constant3/1 -> Add6/1, Product2/2, Product3/2
  Demux1/1 -> Add3/1
  Demux1/2 -> Add3/2
  Add3/1 -> Gain2/1
  Demux1/3 -> Add4/1
  Demux1/4 -> Add4/2
  Add4/1 -> Gain3/1
  Rate Transition3/1 -> Demux1/1
  Gain2/1 -> Saturation Dynamic1/1, Saturation Dynamic/1
  Gain/1 -> Saturation Dynamic1/3, Saturation Dynamic/3
  Saturation Dynamic/1 -> Product/1
  Saturation Dynamic3/1 -> Product3/1
  Saturation Dynamic2/1 -> Product2/1
  Saturation Dynamic1/1 -> Product1/1
  Gain1/1 -> Saturation Dynamic3/3, Saturation Dynamic2/3
  Gain3/1 -> Saturation Dynamic3/1, Saturation Dynamic2/1
  Divide/1 -> Saturation Dynamic3/2, Saturation Dynamic2/2, Saturation Dynamic1/2, Saturation Dynamic/2
  Add5/1 -> Gain4/1
  Saturation1/1 -> Add/1, Divide/1
  Add6/1 -> Divide/2
  Bus Selector1/1 -> MinMax/1, Rate Transition2/1, Rate Transition/1  "<omega>"
  Product4/1 -> Signal Conversion/1, Bus Creator1/1  "M_brems_RF"
  Product5/1 -> Bus Creator1/3, Signal Conversion1/1  "M_brems_RR"
  Gain4/1 -> Add/2
  M_wheel/1 -> Switch/1
  Switch/1 -> Saturation1/1
  input/1 -> Bus Selector1/1
  Gain5/1 -> Divide1/1
  Bus Selector1/2 -> MinMax1/1  "<r_dyn>"
  Constant/1 -> Gain5/1
  MinMax/1 -> Add7/1
  Divide1/1 -> Add7/2
  Add7/1 -> Unit Delay1/1
  Constant1/1 -> Switch/3
  MinMax1/1 -> Divide1/2
  Unit Delay1/1 -> Switch/2
  Bus Selector1/3 -> Dead Zone/1  "<vx>"
  Sign/1 -> Product5/3, Product4/3
  Unit Delay2/1 -> Sign/1
  Dead Zone/1 -> Unit Delay2/1

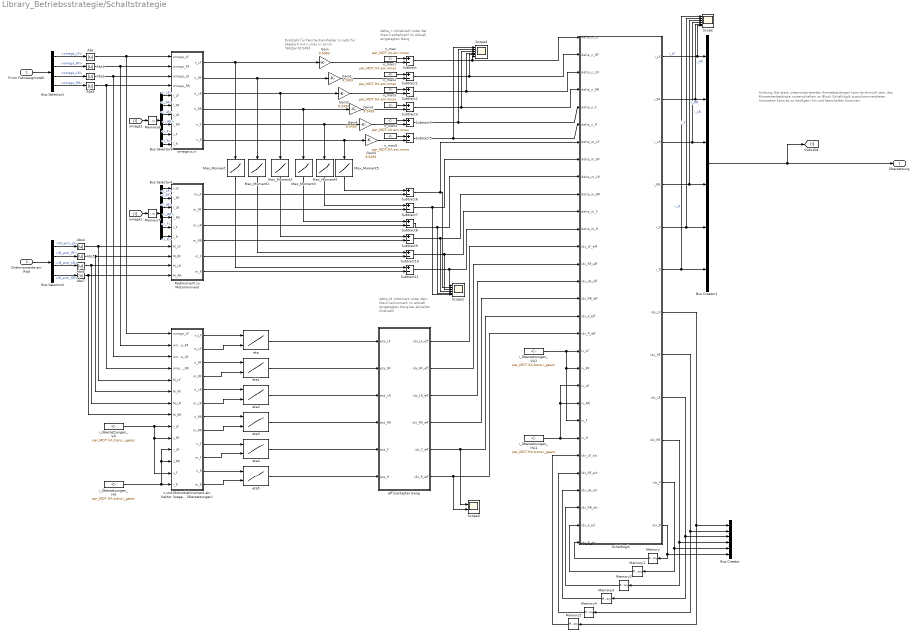
== system Library_Betriebsstrategie/Schaltstrategie ==
  note: delta_n =Drehzahl unter der Maximaldrehzahl im aktuell eingelegten Gang
  note: delta_M =Moment unter dem Maximalmoment im aktuell eingelegten Gang bei aktueller Drehzahl
  note: Achtung: Bei stark untermotorisierten Antriebssträngen kann es sinnvoll sein,
      | das Momentenbedingte runterschalten im Block Schaltlogik auszukommentieren.
      | Ansonsten kann es zu häufigem hin und herschalten kommen.
  note: Drehzahl für Pesche Kennfelder in rad/s
      | für abgleich mit n_max in 1/min
      | *60/2pi=9.5493
  From Fahrzeugmodell : Inport
  Drehmomente am Rad : Inport  Port=2
  Abs{,1..7} (8 alike) : Abs
  Bus Creator : BusCreator  Inputs=6
  Bus Creator1 : BusCreator  Inputs=6
  Bus Selector1 : BusSelector  OutputSignals=omega.omega_LF,omega.omega_RF,omega.omega_LR,omega.omega_RR
  Bus Selector2 : BusSelector  OutputSignals=M_antr_LF,M_antr_RF,M_antr_LR,M_antr_RR
  Bus Selector3 : BusSelector  OutputSignals=i_LF,i_RF,i_LR,i_RR,i_F,i_R
  Bus Selector4 : BusSelector  OutputSignals=i_LF,i_RF,i_LR,i_RR,i_F,i_R
  Gain{,1..5} (6 alike) : Gain  Gain=9.5493
  Max_Moment : Lookup_n-D  NumberOfTableDimensions=1  BreakpointsForDimension1=par_MDT.VA.em.MaxMotorTrqCurve_w  Table=par_MDT.VA.em.MaxMotorTrqCurve_M  InternalRulePriority=Speed  RndMeth=Simplest  InputSameDT=on
  Max_Moment1 : Lookup_n-D  NumberOfTableDimensions=1  BreakpointsForDimension1=par_MDT.VA.em.MaxMotorTrqCurve_w  Table=par_MDT.VA.em.MaxMotorTrqCurve_M  InternalRulePriority=Speed  RndMeth=Simplest  InputSameDT=on
  Max_Moment2 : Lookup_n-D  NumberOfTableDimensions=1  BreakpointsForDimension1=par_MDT.HA.em.MaxMotorTrqCurve_w  Table=par_MDT.HA.em.MaxMotorTrqCurve_M  InternalRulePriority=Speed  RndMeth=Simplest  InputSameDT=on
  Max_Moment3 : Lookup_n-D  NumberOfTableDimensions=1  BreakpointsForDimension1=par_MDT.HA.em.MaxMotorTrqCurve_w  Table=par_MDT.HA.em.MaxMotorTrqCurve_M  InternalRulePriority=Speed  RndMeth=Simplest  InputSameDT=on
  Max_Moment4 : Lookup_n-D  NumberOfTableDimensions=1  BreakpointsForDimension1=par_MDT.VA.em.MaxMotorTrqCurve_w  Table=par_MDT.VA.em.MaxMotorTrqCurve_M  InternalRulePriority=Speed  RndMeth=Simplest  InputSameDT=on
  Max_Moment5 : Lookup_n-D  NumberOfTableDimensions=1  BreakpointsForDimension1=par_MDT.HA.em.MaxMotorTrqCurve_w  Table=par_MDT.HA.em.MaxMotorTrqCurve_M  InternalRulePriority=Speed  RndMeth=Simplest  InputSameDT=on
  Memory{,1..5} (6 alike) : Memory  InitialCondition=1
  Memory6 : Memory
  Memory7 : Memory
  Radmoment zu Motormoment : MATLAB Function  TreatAsAtomicUnit=on
  Schaltlogik : MATLAB Function  TreatAsAtomicUnit=on
  Scope : Scope  NumInputPorts=6
  Scope1 : Scope  NumInputPorts=6
  Scope2 : Scope  NumInputPorts=6
  Scope3 : Scope  NumInputPorts=2
  Subtract{,1..11} (12 alike) : Sum  Inputs=+-
  effizientester Gang : MATLAB Function  TreatAsAtomicUnit=on
  eta : Lookup_n-D  BreakpointsForDimension1=par_MDT.VA.em.MotorEffMap3D_w  BreakpointsForDimension2=par_MDT.VA.em.MotorEffMap3D_M  Table=par_MDT.VA.em.MotorEffMap3D  InternalRulePriority=Speed  RndMeth=Simplest  InputSameDT=on
  eta1 : Lookup_n-D  BreakpointsForDimension1=par_MDT.VA.em.MotorEffMap3D_w  BreakpointsForDimension2=par_MDT.VA.em.MotorEffMap3D_M  Table=par_MDT.VA.em.MotorEffMap3D  InternalRulePriority=Speed  RndMeth=Simplest  InputSameDT=on
  eta2 : Lookup_n-D  BreakpointsForDimension1=par_MDT.HA.em.MotorEffMap3D_w  BreakpointsForDimension2=par_MDT.HA.em.MotorEffMap3D_M  Table=par_MDT.HA.em.MotorEffMap3D  InternalRulePriority=Speed  RndMeth=Simplest  InputSameDT=on
  eta3 : Lookup_n-D  BreakpointsForDimension1=par_MDT.HA.em.MotorEffMap3D_w  BreakpointsForDimension2=par_MDT.HA.em.MotorEffMap3D_M  Table=par_MDT.HA.em.MotorEffMap3D  InternalRulePriority=Speed  RndMeth=Simplest  InputSameDT=on
  eta4 : Lookup_n-D  BreakpointsForDimension1=par_MDT.VA.em.MotorEffMap3D_w  BreakpointsForDimension2=par_MDT.VA.em.MotorEffMap3D_M  Table=par_MDT.VA.em.MotorEffMap3D  InternalRulePriority=Speed  RndMeth=Simplest  InputSameDT=on
  eta5 : Lookup_n-D  BreakpointsForDimension1=par_MDT.HA.em.MotorEffMap3D_w  BreakpointsForDimension2=par_MDT.HA.em.MotorEffMap3D_M  Table=par_MDT.HA.em.MotorEffMap3D  InternalRulePriority=Speed  RndMeth=Simplest  InputSameDT=on
  i_Übersetzungen_HA : Constant  Value=par_MDT.HA.trans.i_gears
  i_Übersetzungen_HA1 : Constant  Value=par_MDT.HA.trans.i_gears
  i_Übersetzungen_VA : Constant  Value=par_MDT.VA.trans.i_gears
  i_Übersetzungen_VA1 : Constant  Value=par_MDT.VA.trans.i_gears
  n und Motordrehmoment als Vektor (wegen ALLEN Übersetzungen) : MATLAB Function  TreatAsAtomicUnit=on
  n_max : Constant  Value=par_MDT.VA.em.nmax
  n_max1 : Constant  Value=par_MDT.VA.em.nmax
  n_max2 : Constant  Value=par_MDT.HA.em.nmax
  n_max3 : Constant  Value=par_MDT.HA.em.nmax
  n_max4 : Constant  Value=par_MDT.VA.em.nmax
  n_max5 : Constant  Value=par_MDT.HA.em.nmax
  omega zu n : MATLAB Function  TreatAsAtomicUnit=on
  Übersetzung : Outport
  wires:
  Gain5/1 -> Subtract5/2
  Gain4/1 -> Subtract4/2
  Gain3/1 -> Subtract3/2
  Gain2/1 -> Subtract2/2
  Gain1/1 -> Subtract1/2
  Gain/1 -> Subtract/2
  i_Übersetzungen_HA1/1 -> Schaltlogik/24(iv_R), Schaltlogik/22(iv_RR), Schaltlogik/21(iv_LR)
  i_Übersetzungen_VA1/1 -> Schaltlogik/19(iv_LF), Schaltlogik/20(iv_RF), Schaltlogik/23(iv_F)
  i_Übersetzungen_HA/1 -> n und Motordrehmoment als Vektor (wegen ALLEN Übersetzungen)/14(i_R), n und Motordrehmoment als Vektor (wegen ALLEN Übersetzungen)/12(i_RR), n und Motordrehmoment als Vektor (wegen ALLEN Übersetzungen)/11(i_LR)
  Bus Selector4/6 -> Radmoment zu Motormoment/6(i_R)  "<i_R>"
  Bus Selector4/5 -> Radmoment zu Motormoment/5(i_F)  "<i_F>"
  Bus Selector4/4 -> Radmoment zu Motormoment/4(i_RR)  "<i_RR>"
  Bus Selector4/3 -> Radmoment zu Motormoment/3(i_LR)  "<i_LR>"
  Bus Selector4/2 -> Radmoment zu Motormoment/2(i_RF)  "<i_RF>"
  Bus Selector4/1 -> Radmoment zu Motormoment/1(i_LF)  "<i_LF>"
  Memory7/1 -> Bus Selector4/1
  [i] -> Memory7/1
  Memory6/1 -> Bus Selector3/1
  Bus Selector3/6 -> omega zu n/10(i_R)  "<i_R>"
  Bus Selector3/5 -> omega zu n/9(i_F)  "<i_F>"
  Bus Selector3/4 -> omega zu n/8(i_RR)  "<i_RR>"
  Bus Selector3/3 -> omega zu n/7(i_LR)  "<i_LR>"
  Bus Selector3/2 -> omega zu n/6(i_RF)  "<i_RF>"
  [i] -> Memory6/1
  Bus Selector3/1 -> omega zu n/5(i_LF)  "<i_LF>"
  Bus Creator1/1 -> Übersetzung/1, [i]
  Schaltlogik/6(i_R) -> Bus Creator1/6, Scope/1  "i_R"
  Schaltlogik/5(i_F) -> Bus Creator1/5, Scope/2  "i_F"
  Schaltlogik/4(i_RR) -> Bus Creator1/4, Scope/3  "i_RR"
  Schaltlogik/3(i_LR) -> Bus Creator1/3, Scope/4  "i_LR"
  Schaltlogik/2(i_RF) -> Bus Creator1/2, Scope/5  "i_RF"
  Schaltlogik/1(i_LF) -> Bus Creator1/1, Scope/6  "i_LF"
  Schaltlogik/10(idx_RR) -> Memory2/1, Bus Creator/4
  Memory5/1 -> Schaltlogik/25(idx_LF_alt)
  Memory4/1 -> Schaltlogik/26(idx_RF_alt)
  Memory3/1 -> Schaltlogik/27(idx_LR_alt)
  Memory2/1 -> Schaltlogik/28(idx_RR_alt)
  Memory1/1 -> Schaltlogik/29(idx_F_alt)
  Memory/1 -> Schaltlogik/30(idx_R_alt)
  Schaltlogik/7(idx_LF) -> Memory5/1, Bus Creator/1
  Schaltlogik/8(idx_RF) -> Memory4/1, Bus Creator/2
  Schaltlogik/9(idx_LR) -> Memory3/1, Bus Creator/3
  Schaltlogik/11(idx_F) -> Memory1/1, Bus Creator/5
  Schaltlogik/12(idx_R) -> Memory/1, Bus Creator/6
  effizientester Gang/6(idx_R_eff) -> Schaltlogik/18(idx_R_eff), Scope3/2
  effizientester Gang/5(idx_F_eff) -> Schaltlogik/17(idx_F_eff), Scope3/1
  effizientester Gang/4(idx_RR_eff) -> Schaltlogik/16(idx_RR_eff)
  effizientester Gang/3(idx_LR_eff) -> Schaltlogik/15(idx_LR_eff)
  effizientester Gang/2(idx_RF_eff) -> Schaltlogik/14(idx_RF_eff)
  effizientester Gang/1(idx_LF_eff) -> Schaltlogik/13(idx_LF_eff)
  Subtract11/1 -> Schaltlogik/12(delta_m_R), Scope1/1
  Subtract10/1 -> Schaltlogik/11(delta_m_F), Scope1/3
  Subtract9/1 -> Schaltlogik/10(delta_m_RR), Scope1/4
  Subtract8/1 -> Schaltlogik/9(delta_m_LR), Scope1/5
  Subtract7/1 -> Schaltlogik/8(delta_m_RF), Scope1/6
  Subtract6/1 -> Schaltlogik/7(delta_m_LF), Scope1/2
  Subtract5/1 -> Schaltlogik/6(delta_n_R), Scope2/1
  Subtract4/1 -> Schaltlogik/5(delta_n_F), Scope2/2
  Subtract3/1 -> Schaltlogik/4(delta_n_RR), Scope2/3
  Subtract2/1 -> Schaltlogik/3(delta_n_LR), Scope2/4
  Subtract1/1 -> Schaltlogik/2(delta_n_RF), Scope2/5
  Subtract/1 -> Schaltlogik/1(delta_n_LF), Scope2/6
  eta5/1 -> effizientester Gang/6(eta_R)
  eta4/1 -> effizientester Gang/5(eta_F)
  eta3/1 -> effizientester Gang/4(eta_RR)
  eta2/1 -> effizientester Gang/3(eta_LR)
  eta1/1 -> effizientester Gang/2(eta_RF)
  eta/1 -> effizientester Gang/1(eta_LF)
  n und Motordrehmoment als Vektor (wegen ALLEN Übersetzungen)/12(m_R) -> eta5/2
  n und Motordrehmoment als Vektor (wegen ALLEN Übersetzungen)/11(n_R) -> eta5/1
  n und Motordrehmoment als Vektor (wegen ALLEN Übersetzungen)/10(m_F) -> eta4/2
  n und Motordrehmoment als Vektor (wegen ALLEN Übersetzungen)/9(n_F) -> eta4/1
  n und Motordrehmoment als Vektor (wegen ALLEN Übersetzungen)/8(m_RR) -> eta3/2
  n und Motordrehmoment als Vektor (wegen ALLEN Übersetzungen)/7(n_RR) -> eta3/1
  n und Motordrehmoment als Vektor (wegen ALLEN Übersetzungen)/6(m_LR) -> eta2/2
  n und Motordrehmoment als Vektor (wegen ALLEN Übersetzungen)/5(n_LR) -> eta2/1
  n und Motordrehmoment als Vektor (wegen ALLEN Übersetzungen)/4(m_RF) -> eta1/2
  n und Motordrehmoment als Vektor (wegen ALLEN Übersetzungen)/3(n_RF) -> eta1/1
  n und Motordrehmoment als Vektor (wegen ALLEN Übersetzungen)/2(m_LF) -> eta/2
  n und Motordrehmoment als Vektor (wegen ALLEN Übersetzungen)/1(n_LF) -> eta/1
  i_Übersetzungen_VA/1 -> n und Motordrehmoment als Vektor (wegen ALLEN Übersetzungen)/9(i_LF), n und Motordrehmoment als Vektor (wegen ALLEN Übersetzungen)/10(i_RF), n und Motordrehmoment als Vektor (wegen ALLEN Übersetzungen)/13(i_F)
  Max_Moment/1 -> Subtract11/1
  Max_Moment1/1 -> Subtract10/1
  Max_Moment2/1 -> Subtract9/1
  Max_Moment3/1 -> Subtract8/1
  Max_Moment4/1 -> Subtract7/1
  Max_Moment5/1 -> Subtract6/1
  Radmoment zu Motormoment/6(m_R) -> Subtract11/2
  Radmoment zu Motormoment/5(m_F) -> Subtract10/2
  Radmoment zu Motormoment/4(m_RR) -> Subtract9/2
  Radmoment zu Motormoment/3(m_LR) -> Subtract8/2
  Radmoment zu Motormoment/2(m_RF) -> Subtract7/2
  Radmoment zu Motormoment/1(m_LF) -> Subtract6/2
  n_max5/1 -> Subtract5/1
  n_max4/1 -> Subtract4/1
  n_max3/1 -> Subtract3/1
  n_max2/1 -> Subtract2/1
  n_max1/1 -> Subtract1/1
  n_max/1 -> Subtract/1
  Bus Selector2/4 -> Abs7/1  "<M_antr_RR>"
  Bus Selector2/3 -> Abs6/1  "<M_antr_LR>"
  Bus Selector2/2 -> Abs5/1  "<M_antr_RF>"
  Bus Selector2/1 -> Abs4/1  "<M_antr_LF>"
  From Fahrzeugmodell/1 -> Bus Selector1/1
  Drehmomente am Rad/1 -> Bus Selector2/1
  Bus Selector1/1 -> Abs/1  "<omega_LF>"
  Bus Selector1/2 -> Abs1/1  "<omega_RF>"
  Bus Selector1/3 -> Abs2/1  "<omega_LR>"
  Bus Selector1/4 -> Abs3/1  "<omega_RR>"
  omega zu n/2(n_RF) -> Gain1/1, Max_Moment1/1
  omega zu n/3(n_LR) -> Gain2/1, Max_Moment2/1
  omega zu n/4(n_RR) -> Gain3/1, Max_Moment3/1
  omega zu n/5(n_F) -> Gain4/1, Max_Moment4/1
  omega zu n/1(n_LF) -> Max_Moment/1, Gain/1
  omega zu n/6(n_R) -> Max_Moment5/1, Gain5/1
  Abs/1 -> omega zu n/1(omega_LF), n und Motordrehmoment als Vektor (wegen ALLEN Übersetzungen)/1(omega_LF)
  Abs1/1 -> omega zu n/2(omega_RF), n und Motordrehmoment als Vektor (wegen ALLEN Übersetzungen)/2(omega_RF)
  Abs2/1 -> omega zu n/3(omega_LR), n und Motordrehmoment als Vektor (wegen ALLEN Übersetzungen)/3(omega_LR)
  Abs3/1 -> omega zu n/4(omega_RR), n und Motordrehmoment als Vektor (wegen ALLEN Übersetzungen)/4(omega_RR)
  Abs4/1 -> Radmoment zu Motormoment/7(M_LF), n und Motordrehmoment als Vektor (wegen ALLEN Übersetzungen)/5(M_LF)
  Abs5/1 -> Radmoment zu Motormoment/8(M_RF), n und Motordrehmoment als Vektor (wegen ALLEN Übersetzungen)/6(M_RF)
  Abs6/1 -> Radmoment zu Motormoment/9(M_LR), n und Motordrehmoment als Vektor (wegen ALLEN Übersetzungen)/7(M_LR)
  Abs7/1 -> Radmoment zu Motormoment/10(M_RR), n und Motordrehmoment als Vektor (wegen ALLEN Übersetzungen)/8(M_RR)

== system Library_Betriebsstrategie/Inverter Power Input einer Achse/Falls radnahe Maschine  ==
  M_achs_EM : Inport
  Constant1 : Constant  Value=az
  Gain : Gain  Gain=0.5
  Switch : Switch  Criteria=u2 > Threshold
  M_mot : Outport
  wires:
  Switch/1 -> M_mot/1
  Gain/1 -> Switch/3
  M_achs_EM/1 -> Gain/1, Switch/1
  Constant1/1 -> Switch/2

== system Library_Betriebsstrategie/Inverter Power Input einer Achse/Falls radnahe Maschine 1 ==
  M_achs_EM : Inport
  Constant1 : Constant  Value=az
  Gain : Gain  Gain=2
  Switch : Switch  Criteria=u2 > Threshold
  M_mot : Outport
  wires:
  Switch/1 -> M_mot/1
  Gain/1 -> Switch/3
  M_achs_EM/1 -> Gain/1, Switch/1
  Constant1/1 -> Switch/2

== system Library_Betriebsstrategie/Inverter Power Input einer Achse/Powerfactorberechnung ==
  Drehmoment : Inport
  Drehzahl : Inport  Port=2
  2-D Lookup Table : Lookup_n-D  BreakpointsForDimension1=torque  BreakpointsForDimension2=speed  Table=Powerfactor_map  ExtrapMethod=Clip  UseLastTableValue=on  InternalRulePriority=Speed  RndMeth=Simplest  InputSameDT=on
  Powerfactor : Outport
  wires:
  Drehmoment/1 -> 2-D Lookup Table/1
  2-D Lookup Table/1 -> Powerfactor/1
  Drehzahl/1 -> 2-D Lookup Table/2

== system Library_Betriebsstrategie/Inverter Power Input einer Achse/Stromberechnung ==
  Leistung : Inport
  Spannung : Inport  Port=2
  Powerfactor : Inport  Port=3
  Constant1 : Constant  Value=3
  Divide : Product  Inputs=*///
  Strom : Outport
  wires:
  Powerfactor/1 -> Divide/4
  Constant1/1 -> Divide/2
  Leistung/1 -> Divide/1
  Spannung/1 -> Divide/3
  Divide/1 -> Strom/1

== system Library_Betriebsstrategie/Inverter Power Input einer Achse/Wirkungsgradberechnung ==
  note: M>0 = 1
  n_mot : Inport
  M_mot : Inport  Port=2
  Add1 : Sum
  Constant : Constant
  Logical Operator : Logic  Operator=NOT  AllPortsSameDT=off  OutDataTypeStr=boolean
  Sign : Signum
  Switch : Switch  Criteria=u2 > Threshold
  generatorischer WKG1 : Subsystem
  motorischer WKG1 : Subsystem
  Wirkungsgrad EM : Outport
  wires:
  Constant/1 -> Add1/1
  Add1/1 -> motorischer WKG1/Enable, Logical Operator/1, Switch/2
  Logical Operator/1 -> generatorischer WKG1/Enable
  Switch/1 -> Wirkungsgrad EM/1
  n_mot/1 -> generatorischer WKG1/1(Drehzahl), motorischer WKG1/1(Drehzahl)
  Sign/1 -> Add1/2
  M_mot/1 -> Sign/1, generatorischer WKG1/2(Moment), motorischer WKG1/2(Moment)
  motorischer WKG1/1(WKG) -> Switch/1
  generatorischer WKG1/1(WKG) -> Switch/3

== system Library_Betriebsstrategie/Inverter Power Input einer Achse/Wirkungsgradberechnung1 ==
  Strom : Inport
  Spannung : Inport  Port=2
  Powerfactor : Inport  Port=3
  n-D Lookup Table : Lookup_n-D  NumberOfTableDimensions=3  BreakpointsForDimension1=current  BreakpointsForDimension2=voltage  BreakpointsForDimension3=powerfactor  Table=efficiency_map_LE  ExtrapMethod=Clip  UseLastTableValue=on  InternalRulePriority=Speed  RndMeth=Simplest  InputSameDT=on
  Wirkungsgrad_LE : Outport
  wires:
  Spannung/1 -> n-D Lookup Table/2
  Powerfactor/1 -> n-D Lookup Table/3
  Strom/1 -> n-D Lookup Table/1
  n-D Lookup Table/1 -> Wirkungsgrad_LE/1

== system Library_Betriebsstrategie/Inverter Power Input einer Achse ALT/Falls radnahe Maschine  ==
  M_achs_EM : Inport
  Constant1 : Constant  Value=az
  Gain : Gain  Gain=0.5
  Switch : Switch  Criteria=u2 > Threshold
  M_mot : Outport
  wires:
  Switch/1 -> M_mot/1
  Gain/1 -> Switch/3
  M_achs_EM/1 -> Gain/1, Switch/1
  Constant1/1 -> Switch/2

== system Library_Betriebsstrategie/Inverter Power Input einer Achse ALT/Leistungselektronik ==
  RMS Spannung : Inport
  Drehmoment_1EM : Inport  Port=2
  "Drehzahl " : Inport  Port=3
  Abs1 : Abs
  Abs2 : Abs
  Abs3 : Abs
  Leistungselektronik : Subsystem
  Powerfactor : Subsystem
  Product1 : Product
  Strom : Subsystem
  Verlustgrad LE : Outport
  wires:
  Abs3/1 -> Powerfactor/2(Drehzahl)
  Abs2/1 -> Powerfactor/1(Drehmoment)
  Product1/1 -> Abs1/1
  "Drehzahl "/1 -> Abs3/1, Product1/2
  Abs1/1 -> Strom/1(Leistung_EM_mech)
  Leistungselektronik/1("Verlustgrad ") -> Verlustgrad LE/1
  Drehmoment_1EM/1 -> Abs2/1, Product1/1
  RMS Spannung/1 -> Strom/2(Spannung), Leistungselektronik/2(Spannung)
  Powerfactor/1(Powerfactor) -> Strom/3(Powerfactor), Leistungselektronik/3(Powerfactor)
  Strom/1(Strom) -> Leistungselektronik/1(Strom)
